simulink model "houseHeating"  (R2024b)
settings: Solver=ode45  StartTime=0.0  StopTime=2500  FixedStep=1  RelTol=1e-3  AbsTol=1e-6
model workspace (MAT data in the model file):
  C = 20
  Cp = 1000
  M = 1778
  Q = 25000
  Req = 0.0015
Description:
  | Thermal Model of a House
  | 
  | This demo illustrates how you can use Simulink(R) to create the thermal model of
  | a house. This system models the outdoor environment, the thermal
  | characteristics of the house, and the house heating system.
  | 
  | The sldemo_househeat_data.m file initializes data in the model workspace.
  | To make changes, you can edit the model workspace directly or edit the MATLAB(R) file
  | and re-load the model workspace.
  | 
  | To view the model workspace, select View > Model Explorer
  | from the Simulink editor.
  | 
  | Note: Time is given in units of hours
settings Model: Creator=The MathWorks, Inc.  LastModifiedBy=sturton
settings SolverCC: AutoScaleAbsTol=off  AlgebraicLoopSolver=TrustRegion
settings DataIOCC: ExternalInput=[]  InitialState=[]
settings OptimizationCC: BlockReduction=off  BooleanDataType=off  ReuseModelBlockBuffer=off  ExpressionDepthLimit=2147483647  InitFltsAndDblsToZero=on  LifeSpan=inf  BufferReusableBoundary=off
settings DebuggingCC: SaveWithParameterizedLinksMsg=none  UnderspecifiedInitializationDetection=Classic  MergeDetectMultiDrivingBlocksExec=none  SignalResolutionControl=TryResolveAllWithWarning  MultiTaskDSMMsg=warning  MultiTaskCondExecSysMsg=none  IntegerOverflowMsg=none  FcnCallInpInsideContextMsg=warning  UnconnectedInputMsg=warning  UnconnectedOutputMsg=warning  UnconnectedLineMsg=warning  BusObjectLabelMismatch=none  StateNameClashWarn=warning  SFUnexpectedBacktrackingDiag=warning  SFNoUnconditionalDefaultTransitionDiag=warning  SFExecutionAtInitializationDiag=none  IntegerSaturationMsg=none  ArithmeticOperatorsInVariantConditions=warning
settings HardwareCC: ProdBitPerPointer=32  ProdBitPerSizeT=32  ProdBitPerPtrDiffT=32  ProdLargestAtomicFloat=None  ProdIntDivRoundTo=Undefined  ProdEndianess=Unspecified  ProdWordSize=32  ProdHWDeviceType=32-bit Generic  TargetUnknown=on
settings ModelReferenceCC: EnableRefExpFcnMdlSchedulingChecks=on  PropagateSignalLabelsOutOfModel=off
settings SFSimCC: SimUseLocalCustomCode=off  CustomCodeUndefinedFunction=UseInterfaceOnly
settings RTWCC: RTWUseLocalCustomCode=off  GPUComputeCapability=3.5
settings CodeAppCC: StateflowObjectComments=on
settings GRTTargetCC: TargetFcnLib=ansi_tfl_tmw.mat  TargetLangStandard=C89/C90 (ANSI)  CombineOutputUpdateFcns=off  GRTInterface=on
settings ConfigComp: CovMetricSettings=dw  CovSaveCumulativeToWorkspaceVar=on  CovSaveSingleToWorkspaceVar=on  CovExternalEMLEnable=off

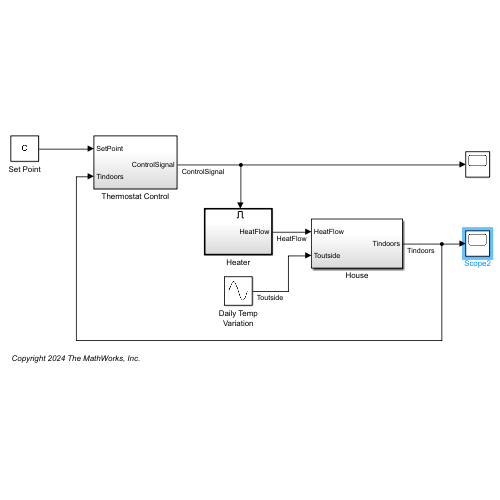
[thumbnail: Simulink's stored preview of the top-level diagram]
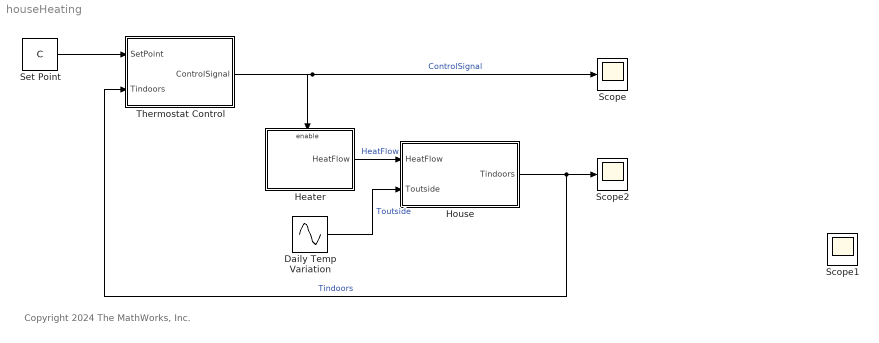
== system houseHeating ==
  note: Copyright 2024 The MathWorks, Inc.
  Daily Temp Variation : Sin  Amplitude=4  Bias=10  Frequency=(2*pi)/(24*3600)  SampleTime=0
  Heater : Subsystem
  House : Subsystem
  Scope : Scope
  Scope2 : Scope
  Set Point : Constant  Value=C
  Thermostat Control : Subsystem
  Scope1 : Scope
  wires:
  House/1(Tindoors) -> Scope2/1, Thermostat Control/2(Tindoors)  "Tindoors"
  Daily Temp Variation/1 -> House/2(Toutside)  "Toutside"
  Heater/1(HeatFlow) -> House/1(HeatFlow)  "HeatFlow"
  Set Point/1 -> Thermostat Control/1(SetPoint)
  Thermostat Control/1(ControlSignal) -> Heater/Enable, Scope/1  "ControlSignal"

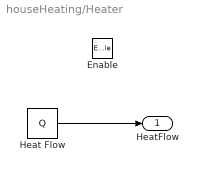
== system houseHeating/Heater ==
  Enable : EnablePort
  Heat Flow : Constant  Value=Q
  HeatFlow : Outport  OutputWhenDisabled=reset  InitialOutput=0
  wires:
  Heat Flow/1 -> HeatFlow/1

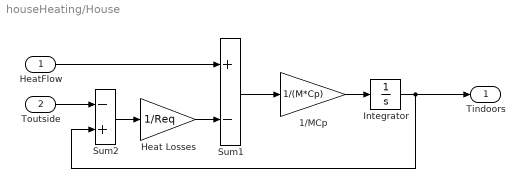
== system houseHeating/House ==
  HeatFlow : Inport
  Toutside : Inport  Port=2
  1/MCp : Gain  Gain=1/(M*Cp)  SaturateOnIntegerOverflow=on  OutDataTypeStr=Inherit: Same as input  ParamDataTypeStr=Inherit: Same as input
  Heat Losses : Gain  Gain=1/Req  SaturateOnIntegerOverflow=on  OutDataTypeStr=Inherit: Same as input  ParamDataTypeStr=Inherit: Same as input
  Integrator : Integrator  InitialCondition=18
  Sum1 : Sum  Inputs=+-  InputSameDT=on  SaturateOnIntegerOverflow=on  OutDataTypeStr=Inherit: Same as first input
  Sum2 : Sum  Inputs=-+  InputSameDT=on  SaturateOnIntegerOverflow=on  OutDataTypeStr=Inherit: Same as first input
  Tindoors : Outport  InitialOutput=0  VectorParamsAs1DForOutWhenUnconnected=off
  wires:
  Toutside/1 -> Sum2/1
  HeatFlow/1 -> Sum1/1
  Sum1/1 -> 1/MCp/1
  Sum2/1 -> Heat Losses/1
  Heat Losses/1 -> Sum1/2
  1/MCp/1 -> Integrator/1
  Integrator/1 -> Tindoors/1, Sum2/2

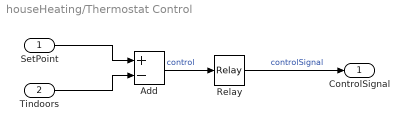
== system houseHeating/Thermostat Control ==
  SetPoint : Inport
  Tindoors : Inport  Port=2
  Add : Sum  Inputs=+-
  Relay : Relay  OnSwitchValue=1  OffSwitchValue=-1
  ControlSignal : Outport
  wires:
  Add/1 -> Relay/1  "control"
  Tindoors/1 -> Add/2
  SetPoint/1 -> Add/1
  Relay/1 -> ControlSignal/1  "controlSignal"
